simulink model "FuzzyPD_2DOFRobot"  (R2024b)
settings: Solver=FixedStepAuto  StartTime=0.0  StopTime=40.0  FixedStep=0.01  RelTol=1e-3
libraries: neural x58
(part 2 of 2)

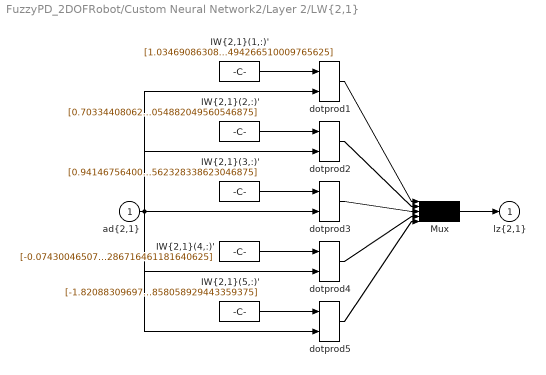
== system FuzzyPD_2DOFRobot/Custom Neural Network2/Layer 2/LW{2,1} ==
  "ad{2,1}" : Inport  PortDimensions=20
      mask Display: e = 0.06;c1 = [120 230 180]/255;c2 = ([120 230 180]+0)/(256+128);c3 = ([120 230 180]+128)/(256+128);patch([0 1 1 0],[0 0 1 1],c1);patch([0 1 1 1-e 1-e 0+e],[0 0 1 1-e 0+e 0+e],c2);patch([0 0 1 1-e 0+e 0+e],[0 1 1 1-e 1-e 0+e],c3);plot([0 1 1 0 0],[0 0 1 1 0]);
  "IW{2,1}(1,:)'" : Constant  Value=[1.034690863083454370752178874681703746318817138671875;0.71478762496765357870032175924279727041721343994140625;-0.9023035135599835054875939022167585790157318115234375;0.433374758147354099957482276295195333659648895263671875;1.2128826774850207659284251349163241684436798095703125;-0.028405390176671818647236023025470785796642303466796875;-0.80937341754777836211331987215089611709117889404296875;-0.545930474311120850217093902756460011005401611328125;0.8748460535361985979108112587709911167621612548828125;0.67782045911715138597486429716809652745723724365234375;-1.0204186771718684045850977781810797750949859619140625;-1.05206299588309892811821555369533598423004150390625;-0.853743879382991455173623762675561010837554931640625;0.860297114781614080669669419876299798488616943359375;1.484280086079977412083508170326240360736846923828125;0.58045414384198534829550908398232422769069671630859375;-0.052367665752894927699845339930107002146542072296142578125;0.2329001374967674120597393994103185832500457763671875;0.772776795739658073358668843866325914859771728515625;-0.58307313814202521573548665401176549494266510009765625]
      mask Display: e = 0.06;c1 = [120 150 230]/255;c2 = ([120 150 230]+0)/383;c3 = ([120 150 230]+128)/383;patch([0 1 1 0],[0 0 1 1],c1);patch([0 1 1 1-e 1-e 0+e],[0 0 1 1-e 0+e 0+e],c2);patch([0 0 1 1-e 0+e 0+e],[0 1 1 1-e 1-e 0+e],c3);plot([0 1 1 0 0],[0 0 1 1 0]);disp('weights');
  "IW{2,1}(2,:)'" : Constant  Value=[0.70334408062744924183817829543841071426868438720703125;-0.53939593820879061514261820775573141872882843017578125;1.137406415460587627563882051617838442325592041015625;-0.4474318401098182906849842765950597822666168212890625;1.6403418277065695551897306359023787081241607666015625;-0.62450917338377631704560144498827867209911346435546875;1.4154537351861751215409412907320074737071990966796875;0.370117096077064722248195494103129021823406219482421875;-1.4599460757945610378527590000885538756847381591796875;1.24160115883402877301477928995154798030853271484375;-0.560063640244826910219444471294991672039031982421875;-0.44157853574027561283088516574935056269168853759765625;0.638904752277584808695110041298903524875640869140625;-0.298521682975893931644151280124788172543048858642578125;1.134156749895475879696959964348934590816497802734375;0.533255671669086606101473080343566834926605224609375;-0.6331474081832733080688058180385269224643707275390625;-1.0542382294758991800875946864834986627101898193359375;-0.43008412156374575818773564606090076267719268798828125;-1.6039047144127873689711805127444677054882049560546875]
      mask Display: e = 0.06;c1 = [120 150 230]/255;c2 = ([120 150 230]+0)/383;c3 = ([120 150 230]+128)/383;patch([0 1 1 0],[0 0 1 1],c1);patch([0 1 1 1-e 1-e 0+e],[0 0 1 1-e 0+e 0+e],c2);patch([0 0 1 1-e 0+e 0+e],[0 1 1 1-e 1-e 0+e],c3);plot([0 1 1 0 0],[0 0 1 1 0]);disp('weights');
  "IW{2,1}(3,:)'" : Constant  Value=[0.94146756400392683783451275303377769887447357177734375;0.4731251034591033022280726072494871914386749267578125;0.352835011006732146565667562754242680966854095458984375;0.83254717249503784604058864715625531971454620361328125;0.3824725814911185128863735371851362287998199462890625;-0.6642082095069279379373483607196249067783355712890625;-0.6011230376676464093321783366263844072818756103515625;0.7943446655054771099457866512238979339599609375;-0.272249257525836119153694880878902040421962738037109375;0.43212706390093968966681359233916737139225006103515625;-0.7383066341177497715619892915128730237483978271484375;-0.366647708417497997235301454566069878637790679931640625;-0.71722827145524148395594465910107828676700592041015625;0.95313490510591158955122637053136713802814483642578125;0.1959390264021163563512573091429658234119415283203125;-0.59216619609386622613556028227321803569793701171875;0.837133704178429471909339554258622229099273681640625;-0.95864630287372076811180932054412551224231719970703125;0.9581049364333307227781233450514264404773712158203125;0.852489248366903762388346876832656562328338623046875]
      mask Display: e = 0.06;c1 = [120 150 230]/255;c2 = ([120 150 230]+0)/383;c3 = ([120 150 230]+128)/383;patch([0 1 1 0],[0 0 1 1],c1);patch([0 1 1 1-e 1-e 0+e],[0 0 1 1-e 0+e 0+e],c2);patch([0 0 1 1-e 0+e 0+e],[0 1 1 1-e 1-e 0+e],c3);plot([0 1 1 0 0],[0 0 1 1 0]);disp('weights');
  "IW{2,1}(4,:)'" : Constant  Value=[-0.07430046507749595019465260747892898507416248321533203125;-0.98614127796260497849090143063222058117389678955078125;0.058465987251093365362208942315191961824893951416015625;0.55693630778370117884179535394650883972644805908203125;0.9257628102854227325479996579815633594989776611328125;-0.72377518289734277256997074800892733037471771240234375;2.023327190999340441379672483890317380428314208984375;-0.330409569161653371427433967255637980997562408447265625;1.2305003744543070443029364469111897051334381103515625;1.409296668044323297408482176251709461212158203125;-0.8464601958773758649812180010485462844371795654296875;-0.15917964775082149575524681495153345167636871337890625;0.022421149902434732437139786043189815245568752288818359375;-1.4635363788993991374098868618602864444255828857421875;0.37541953637812941479978690040297806262969970703125;2.088562987566513928783251685672439634799957275390625;0.47790382938157727199524060779367573559284210205078125;-1.81498933367571613217705817078240215778350830078125;0.337827387873957663000368256689398549497127532958984375;-0.2216054912450064195983401305056759156286716461181640625]
      mask Display: e = 0.06;c1 = [120 150 230]/255;c2 = ([120 150 230]+0)/383;c3 = ([120 150 230]+128)/383;patch([0 1 1 0],[0 0 1 1],c1);patch([0 1 1 1-e 1-e 0+e],[0 0 1 1-e 0+e 0+e],c2);patch([0 0 1 1-e 0+e 0+e],[0 1 1 1-e 1-e 0+e],c3);plot([0 1 1 0 0],[0 0 1 1 0]);disp('weights');
  "IW{2,1}(5,:)'" : Constant  Value=[-1.8208830969722242798525257967412471771240234375;0.69084466334677185894719286807230673730373382568359375;1.122947859773492762514024434494785964488983154296875;-0.317234295989334114107549567052046768367290496826171875;0.62250476604156224080810488885617814958095550537109375;1.6894068695845165795077491566189564764499664306640625;0.288506114882021658107902339907013811171054840087890625;0.58551374156033630935525025051902048289775848388671875;0.6922866926558828293281067089992575347423553466796875;0.6889586364774105131658643585979007184505462646484375;-0.432375825434855531881339629762805998325347900390625;0.097155559921801526446216712429304607212543487548828125;-1.6078115193098370117041895355214364826679229736328125;0.08076992178353738227603031418766477145254611968994140625;0.284325215938594222375712661232682876288890838623046875;2.95425971495564443358716744114644825458526611328125;-1.4133445517274896285897511916118673980236053466796875;-1.9814217989859825852505537113756872713565826416015625;0.98014144968227956411510604084469377994537353515625;-4.094403814209552905367672792635858058929443359375]
      mask Display: e = 0.06;c1 = [120 150 230]/255;c2 = ([120 150 230]+0)/383;c3 = ([120 150 230]+128)/383;patch([0 1 1 0],[0 0 1 1],c1);patch([0 1 1 1-e 1-e 0+e],[0 0 1 1-e 0+e 0+e],c2);patch([0 0 1 1-e 0+e 0+e],[0 1 1 1-e 1-e 0+e],c3);plot([0 1 1 0 0],[0 0 1 1 0]);disp('weights');
  Mux : Mux  Inputs=5
      mask Display: e = 0.06;c1 = [120 150 230]/255;c2 = ([120 150 230]+0)/383;c3 = ([120 150 230]+128)/383;patch([0 1 1 0],[0 0 1 1],c1);patch([0 1 1 1-e 1-e 0+e],[0 0 1 1-e 0+e 0+e],c2);patch([0 0 1 1-e 0+e 0+e],[0 1 1 1-e 1-e 0+e],c3);plot([0 1 1 0 0],[0 0 1 1 0]);disp('Mux');
  dotprod{1..5} (5 alike) : neural/Weight Functions/dotprod
  "lz{2,1}" : Outport
      mask Display: e = 0.06;c1 = [120 230 180]/255;c2 = ([120 230 180]+0)/(256+128);c3 = ([120 230 180]+128)/(256+128);patch([0 1 1 0],[0 0 1 1],c1);patch([0 1 1 1-e 1-e 0+e],[0 0 1 1-e 0+e 0+e],c2);patch([0 0 1 1-e 0+e 0+e],[0 1 1 1-e 1-e 0+e],c3);plot([0 1 1 0 0],[0 0 1 1 0]);
  wires:
  "IW{2,1}(1,:)'"/1 -> dotprod1/1
  "ad{2,1}"/1 -> dotprod1/2, dotprod2/2, dotprod3/2, dotprod4/2, dotprod5/2
  dotprod1/1 -> Mux/1
  "IW{2,1}(2,:)'"/1 -> dotprod2/1
  dotprod2/1 -> Mux/2
  "IW{2,1}(3,:)'"/1 -> dotprod3/1
  dotprod3/1 -> Mux/3
  "IW{2,1}(4,:)'"/1 -> dotprod4/1
  dotprod4/1 -> Mux/4
  "IW{2,1}(5,:)'"/1 -> dotprod5/1
  dotprod5/1 -> Mux/5
  Mux/1 -> "lz{2,1}"/1

== system FuzzyPD_2DOFRobot/Custom Neural Network2/Layer 3/Delays 1 ==
  "p{3}" : Inport  PortDimensions=5
      mask Display: e = 0.06;c1 = [120 230 180]/255;c2 = ([120 230 180]+0)/(256+128);c3 = ([120 230 180]+128)/(256+128);patch([0 1 1 0],[0 0 1 1],c1);patch([0 1 1 1-e 1-e 0+e],[0 0 1 1-e 0+e 0+e],c2);patch([0 0 1 1-e 0+e 0+e],[0 1 1 1-e 1-e 0+e],c3);plot([0 1 1 0 0],[0 0 1 1 0]);
  mux : Mux  Inputs=1
      mask Display: e = 0.06;c1 = [120 150 230]/255;c2 = ([120 150 230]+0)/383;c3 = ([120 150 230]+128)/383;patch([0 1 1 0],[0 0 1 1],c1);patch([0 1 1 1-e 1-e 0+e],[0 0 1 1-e 0+e 0+e],c2);patch([0 0 1 1-e 0+e 0+e],[0 1 1 1-e 1-e 0+e],c3);plot([0 1 1 0 0],[0 0 1 1 0]);disp('Mux')
  "pd{3,2}" : Outport
      mask Display: e = 0.06;c1 = [120 230 180]/255;c2 = ([120 230 180]+0)/(256+128);c3 = ([120 230 180]+128)/(256+128);patch([0 1 1 0],[0 0 1 1],c1);patch([0 1 1 1-e 1-e 0+e],[0 0 1 1-e 0+e 0+e],c2);patch([0 0 1 1-e 0+e 0+e],[0 1 1 1-e 1-e 0+e],c3);plot([0 1 1 0 0],[0 0 1 1 0]);
  wires:
  "p{3}"/1 -> mux/1
  mux/1 -> "pd{3,2}"/1

== system FuzzyPD_2DOFRobot/Custom Neural Network2/Layer 3/LW{3,2} ==
  "ad{3,2}" : Inport  PortDimensions=5
      mask Display: e = 0.06;c1 = [120 230 180]/255;c2 = ([120 230 180]+0)/(256+128);c3 = ([120 230 180]+128)/(256+128);patch([0 1 1 0],[0 0 1 1],c1);patch([0 1 1 1-e 1-e 0+e],[0 0 1 1-e 0+e 0+e],c2);patch([0 0 1 1-e 0+e 0+e],[0 1 1 1-e 1-e 0+e],c3);plot([0 1 1 0 0],[0 0 1 1 0]);
  "IW{3,2}(1,:)'" : Constant  Value=[1.7210370476344756252018441955442540347576141357421875;0.96563713038743392846896540504531003534793853759765625;0.6139936572474160580981106249964796006679534912109375;1.4959984213294006405448044461081735789775848388671875;0.600176864765051387706762398011051118373870849609375]
      mask Display: e = 0.06;c1 = [120 150 230]/255;c2 = ([120 150 230]+0)/383;c3 = ([120 150 230]+128)/383;patch([0 1 1 0],[0 0 1 1],c1);patch([0 1 1 1-e 1-e 0+e],[0 0 1 1-e 0+e 0+e],c2);patch([0 0 1 1-e 0+e 0+e],[0 1 1 1-e 1-e 0+e],c3);plot([0 1 1 0 0],[0 0 1 1 0]);disp('weights');
  Mux : Mux  Inputs=1
      mask Display: e = 0.06;c1 = [120 150 230]/255;c2 = ([120 150 230]+0)/383;c3 = ([120 150 230]+128)/383;patch([0 1 1 0],[0 0 1 1],c1);patch([0 1 1 1-e 1-e 0+e],[0 0 1 1-e 0+e 0+e],c2);patch([0 0 1 1-e 0+e 0+e],[0 1 1 1-e 1-e 0+e],c3);plot([0 1 1 0 0],[0 0 1 1 0]);disp('Mux');
  dotprod1 : neural/Weight Functions/dotprod
  "lz{3,2}" : Outport
      mask Display: e = 0.06;c1 = [120 230 180]/255;c2 = ([120 230 180]+0)/(256+128);c3 = ([120 230 180]+128)/(256+128);patch([0 1 1 0],[0 0 1 1],c1);patch([0 1 1 1-e 1-e 0+e],[0 0 1 1-e 0+e 0+e],c2);patch([0 0 1 1-e 0+e 0+e],[0 1 1 1-e 1-e 0+e],c3);plot([0 1 1 0 0],[0 0 1 1 0]);
  wires:
  "IW{3,2}(1,:)'"/1 -> dotprod1/1
  "ad{3,2}"/1 -> dotprod1/2
  dotprod1/1 -> Mux/1
  Mux/1 -> "lz{3,2}"/1

== system FuzzyPD_2DOFRobot/Custom Neural Network3/Layer 1/Delays 1 ==
  "p{1}" : Inport  PortDimensions=3
      mask Display: e = 0.06;c1 = [120 230 180]/255;c2 = ([120 230 180]+0)/(256+128);c3 = ([120 230 180]+128)/(256+128);patch([0 1 1 0],[0 0 1 1],c1);patch([0 1 1 1-e 1-e 0+e],[0 0 1 1-e 0+e 0+e],c2);patch([0 0 1 1-e 0+e 0+e],[0 1 1 1-e 1-e 0+e],c3);plot([0 1 1 0 0],[0 0 1 1 0]);
  mux : Mux  Inputs=1
      mask Display: e = 0.06;c1 = [120 150 230]/255;c2 = ([120 150 230]+0)/383;c3 = ([120 150 230]+128)/383;patch([0 1 1 0],[0 0 1 1],c1);patch([0 1 1 1-e 1-e 0+e],[0 0 1 1-e 0+e 0+e],c2);patch([0 0 1 1-e 0+e 0+e],[0 1 1 1-e 1-e 0+e],c3);plot([0 1 1 0 0],[0 0 1 1 0]);disp('Mux')
  "pd{1,1}" : Outport
      mask Display: e = 0.06;c1 = [120 230 180]/255;c2 = ([120 230 180]+0)/(256+128);c3 = ([120 230 180]+128)/(256+128);patch([0 1 1 0],[0 0 1 1],c1);patch([0 1 1 1-e 1-e 0+e],[0 0 1 1-e 0+e 0+e],c2);patch([0 0 1 1-e 0+e 0+e],[0 1 1 1-e 1-e 0+e],c3);plot([0 1 1 0 0],[0 0 1 1 0]);
  wires:
  "p{1}"/1 -> mux/1
  mux/1 -> "pd{1,1}"/1

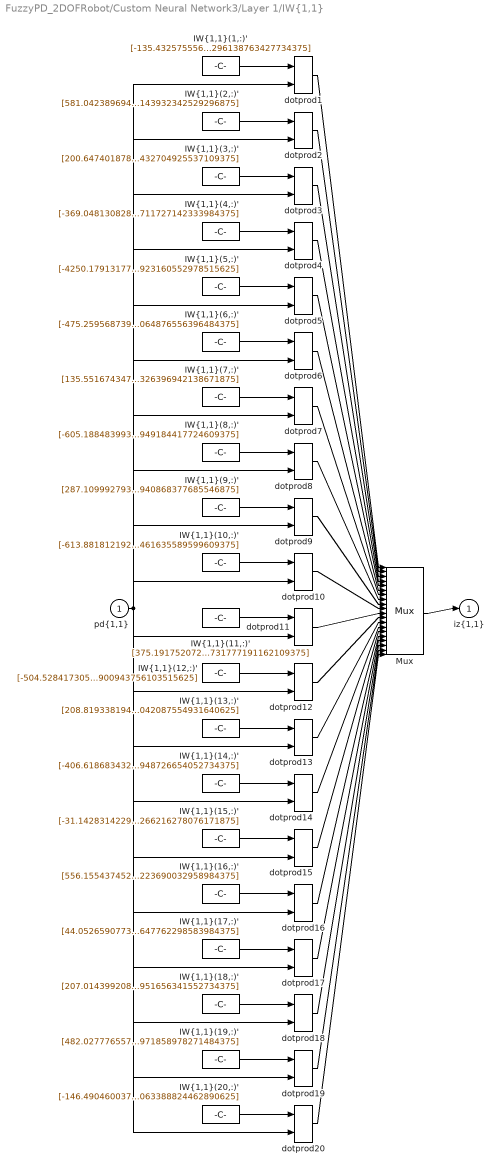
== system FuzzyPD_2DOFRobot/Custom Neural Network3/Layer 1/IW{1,1} ==
  "pd{1,1}" : Inport  PortDimensions=3
      mask Display: e = 0.06;c1 = [120 230 180]/255;c2 = ([120 230 180]+0)/(256+128);c3 = ([120 230 180]+128)/(256+128);patch([0 1 1 0],[0 0 1 1],c1);patch([0 1 1 1-e 1-e 0+e],[0 0 1 1-e 0+e 0+e],c2);patch([0 0 1 1-e 0+e 0+e],[0 1 1 1-e 1-e 0+e],c3);plot([0 1 1 0 0],[0 0 1 1 0]);
  "IW{1,1}(1,:)'" : Constant  Value=[-135.432575556479292799849645234644412994384765625;10.0754622663960358153190099983476102352142333984375;-0.472792983898389473917944769709720276296138763427734375]
      mask Display: e = 0.06;c1 = [120 150 230]/255;c2 = ([120 150 230]+0)/383;c3 = ([120 150 230]+128)/383;patch([0 1 1 0],[0 0 1 1],c1);patch([0 1 1 1-e 1-e 0+e],[0 0 1 1-e 0+e 0+e],c2);patch([0 0 1 1-e 0+e 0+e],[0 1 1 1-e 1-e 0+e],c3);plot([0 1 1 0 0],[0 0 1 1 0]);disp('Weights');
  "IW{1,1}(10,:)'" : Constant  Value=[-613.881812192461666199960745871067047119140625;94.37434568259828893133089877665042877197265625;0.2210466396896054452891888786325580440461635589599609375]
      mask Display: e = 0.06;c1 = [120 150 230]/255;c2 = ([120 150 230]+0)/383;c3 = ([120 150 230]+128)/383;patch([0 1 1 0],[0 0 1 1],c1);patch([0 1 1 1-e 1-e 0+e],[0 0 1 1-e 0+e 0+e],c2);patch([0 0 1 1-e 0+e 0+e],[0 1 1 1-e 1-e 0+e],c3);plot([0 1 1 0 0],[0 0 1 1 0]);disp('Weights');
  "IW{1,1}(11,:)'" : Constant  Value=[375.19175207238521352337556891143321990966796875;-30.256984409509783517933101393282413482666015625;-0.10059679238582529270384924302561557851731777191162109375]
      mask Display: e = 0.06;c1 = [120 150 230]/255;c2 = ([120 150 230]+0)/383;c3 = ([120 150 230]+128)/383;patch([0 1 1 0],[0 0 1 1],c1);patch([0 1 1 1-e 1-e 0+e],[0 0 1 1-e 0+e 0+e],c2);patch([0 0 1 1-e 0+e 0+e],[0 1 1 1-e 1-e 0+e],c3);plot([0 1 1 0 0],[0 0 1 1 0]);disp('Weights');
  "IW{1,1}(12,:)'" : Constant  Value=[-504.52841730549317844634060747921466827392578125;7.89932038819319615186032024212181568145751953125;-0.07291021612746741153987528605284751392900943756103515625]
      mask Display: e = 0.06;c1 = [120 150 230]/255;c2 = ([120 150 230]+0)/383;c3 = ([120 150 230]+128)/383;patch([0 1 1 0],[0 0 1 1],c1);patch([0 1 1 1-e 1-e 0+e],[0 0 1 1-e 0+e 0+e],c2);patch([0 0 1 1-e 0+e 0+e],[0 1 1 1-e 1-e 0+e],c3);plot([0 1 1 0 0],[0 0 1 1 0]);disp('Weights');
  "IW{1,1}(13,:)'" : Constant  Value=[208.819338194989853718652739189565181732177734375;37.72759958928005374900749302469193935394287109375;-0.757522513115136408856642447062768042087554931640625]
      mask Display: e = 0.06;c1 = [120 150 230]/255;c2 = ([120 150 230]+0)/383;c3 = ([120 150 230]+128)/383;patch([0 1 1 0],[0 0 1 1],c1);patch([0 1 1 1-e 1-e 0+e],[0 0 1 1-e 0+e 0+e],c2);patch([0 0 1 1-e 0+e 0+e],[0 1 1 1-e 1-e 0+e],c3);plot([0 1 1 0 0],[0 0 1 1 0]);disp('Weights');
  "IW{1,1}(14,:)'" : Constant  Value=[-406.61868343285050286795012652873992919921875;-24.0765119392089701477743801660835742950439453125;-0.9332100225159842832312051541521213948726654052734375]
      mask Display: e = 0.06;c1 = [120 150 230]/255;c2 = ([120 150 230]+0)/383;c3 = ([120 150 230]+128)/383;patch([0 1 1 0],[0 0 1 1],c1);patch([0 1 1 1-e 1-e 0+e],[0 0 1 1-e 0+e 0+e],c2);patch([0 0 1 1-e 0+e 0+e],[0 1 1 1-e 1-e 0+e],c3);plot([0 1 1 0 0],[0 0 1 1 0]);disp('Weights');
  "IW{1,1}(15,:)'" : Constant  Value=[-31.142831422933721086110381293110549449920654296875;5.93410486604341347316449173376895487308502197265625;0.335283700642425130933332866334239952266216278076171875]
      mask Display: e = 0.06;c1 = [120 150 230]/255;c2 = ([120 150 230]+0)/383;c3 = ([120 150 230]+128)/383;patch([0 1 1 0],[0 0 1 1],c1);patch([0 1 1 1-e 1-e 0+e],[0 0 1 1-e 0+e 0+e],c2);patch([0 0 1 1-e 0+e 0+e],[0 1 1 1-e 1-e 0+e],c3);plot([0 1 1 0 0],[0 0 1 1 0]);disp('Weights');
  "IW{1,1}(16,:)'" : Constant  Value=[556.15543745200511693838052451610565185546875;-62.75604466827012828389342757873237133026123046875;0.98338532426563973753985692383139394223690032958984375]
      mask Display: e = 0.06;c1 = [120 150 230]/255;c2 = ([120 150 230]+0)/383;c3 = ([120 150 230]+128)/383;patch([0 1 1 0],[0 0 1 1],c1);patch([0 1 1 1-e 1-e 0+e],[0 0 1 1-e 0+e 0+e],c2);patch([0 0 1 1-e 0+e 0+e],[0 1 1 1-e 1-e 0+e],c3);plot([0 1 1 0 0],[0 0 1 1 0]);disp('Weights');
  "IW{1,1}(17,:)'" : Constant  Value=[44.05265907730446173218297190032899379730224609375;-23.092237387069513232518147560767829418182373046875;0.94364919863966834068236266830353997647762298583984375]
      mask Display: e = 0.06;c1 = [120 150 230]/255;c2 = ([120 150 230]+0)/383;c3 = ([120 150 230]+128)/383;patch([0 1 1 0],[0 0 1 1],c1);patch([0 1 1 1-e 1-e 0+e],[0 0 1 1-e 0+e 0+e],c2);patch([0 0 1 1-e 0+e 0+e],[0 1 1 1-e 1-e 0+e],c3);plot([0 1 1 0 0],[0 0 1 1 0]);disp('Weights');
  "IW{1,1}(18,:)'" : Constant  Value=[207.014399208383252926068962551653385162353515625;-10.5004037937094931720594104263000190258026123046875;0.049000063312716966856807943031526519916951656341552734375]
      mask Display: e = 0.06;c1 = [120 150 230]/255;c2 = ([120 150 230]+0)/383;c3 = ([120 150 230]+128)/383;patch([0 1 1 0],[0 0 1 1],c1);patch([0 1 1 1-e 1-e 0+e],[0 0 1 1-e 0+e 0+e],c2);patch([0 0 1 1-e 0+e 0+e],[0 1 1 1-e 1-e 0+e],c3);plot([0 1 1 0 0],[0 0 1 1 0]);disp('Weights');
  "IW{1,1}(19,:)'" : Constant  Value=[482.02777655767641817874391563236713409423828125;15.4991899483087092193045464227907359600067138671875;-0.349070997444174524471094400723814032971858978271484375]
      mask Display: e = 0.06;c1 = [120 150 230]/255;c2 = ([120 150 230]+0)/383;c3 = ([120 150 230]+128)/383;patch([0 1 1 0],[0 0 1 1],c1);patch([0 1 1 1-e 1-e 0+e],[0 0 1 1-e 0+e 0+e],c2);patch([0 0 1 1-e 0+e 0+e],[0 1 1 1-e 1-e 0+e],c3);plot([0 1 1 0 0],[0 0 1 1 0]);disp('Weights');
  "IW{1,1}(2,:)'" : Constant  Value=[581.0423896949167783532175235450267791748046875;16.47915141783929726670976378954946994781494140625;0.466023100877216822635062953850138001143932342529296875]
      mask Display: e = 0.06;c1 = [120 150 230]/255;c2 = ([120 150 230]+0)/383;c3 = ([120 150 230]+128)/383;patch([0 1 1 0],[0 0 1 1],c1);patch([0 1 1 1-e 1-e 0+e],[0 0 1 1-e 0+e 0+e],c2);patch([0 0 1 1-e 0+e 0+e],[0 1 1 1-e 1-e 0+e],c3);plot([0 1 1 0 0],[0 0 1 1 0]);disp('Weights');
  "IW{1,1}(20,:)'" : Constant  Value=[-146.490460037200847409621928818523883819580078125;65.6835974049690776155330240726470947265625;0.060311156693250246585424889644855284132063388824462890625]
      mask Display: e = 0.06;c1 = [120 150 230]/255;c2 = ([120 150 230]+0)/383;c3 = ([120 150 230]+128)/383;patch([0 1 1 0],[0 0 1 1],c1);patch([0 1 1 1-e 1-e 0+e],[0 0 1 1-e 0+e 0+e],c2);patch([0 0 1 1-e 0+e 0+e],[0 1 1 1-e 1-e 0+e],c3);plot([0 1 1 0 0],[0 0 1 1 0]);disp('Weights');
  "IW{1,1}(3,:)'" : Constant  Value=[200.647401878155420718030654825270175933837890625;32.5421531128873340321661089546978473663330078125;0.385099895085624088775233531123376451432704925537109375]
      mask Display: e = 0.06;c1 = [120 150 230]/255;c2 = ([120 150 230]+0)/383;c3 = ([120 150 230]+128)/383;patch([0 1 1 0],[0 0 1 1],c1);patch([0 1 1 1-e 1-e 0+e],[0 0 1 1-e 0+e 0+e],c2);patch([0 0 1 1-e 0+e 0+e],[0 1 1 1-e 1-e 0+e],c3);plot([0 1 1 0 0],[0 0 1 1 0]);disp('Weights');
  "IW{1,1}(4,:)'" : Constant  Value=[-369.04813082858544248665566556155681610107421875;2.229120603719899396111259193276055157184600830078125;-0.27087284001736777749869133913307450711727142333984375]
      mask Display: e = 0.06;c1 = [120 150 230]/255;c2 = ([120 150 230]+0)/383;c3 = ([120 150 230]+128)/383;patch([0 1 1 0],[0 0 1 1],c1);patch([0 1 1 1-e 1-e 0+e],[0 0 1 1-e 0+e 0+e],c2);patch([0 0 1 1-e 0+e 0+e],[0 1 1 1-e 1-e 0+e],c3);plot([0 1 1 0 0],[0 0 1 1 0]);disp('Weights');
  "IW{1,1}(5,:)'" : Constant  Value=[-4250.179131777787915780209004878997802734375;21.35109343006629245564909069798886775970458984375;-0.9095295811207879665971631766296923160552978515625]
      mask Display: e = 0.06;c1 = [120 150 230]/255;c2 = ([120 150 230]+0)/383;c3 = ([120 150 230]+128)/383;patch([0 1 1 0],[0 0 1 1],c1);patch([0 1 1 1-e 1-e 0+e],[0 0 1 1-e 0+e 0+e],c2);patch([0 0 1 1-e 0+e 0+e],[0 1 1 1-e 1-e 0+e],c3);plot([0 1 1 0 0],[0 0 1 1 0]);disp('Weights');
  "IW{1,1}(6,:)'" : Constant  Value=[-475.25956873974388372516841627657413482666015625;-38.50212833135109491422554128803312778472900390625;1.2676270783202507885789600550197064876556396484375]
      mask Display: e = 0.06;c1 = [120 150 230]/255;c2 = ([120 150 230]+0)/383;c3 = ([120 150 230]+128)/383;patch([0 1 1 0],[0 0 1 1],c1);patch([0 1 1 1-e 1-e 0+e],[0 0 1 1-e 0+e 0+e],c2);patch([0 0 1 1-e 0+e 0+e],[0 1 1 1-e 1-e 0+e],c3);plot([0 1 1 0 0],[0 0 1 1 0]);disp('Weights');
  "IW{1,1}(7,:)'" : Constant  Value=[135.551674347247882224110071547329425811767578125;-192.756809317032320905127562582492828369140625;0.1987756467040510954813470334556768648326396942138671875]
      mask Display: e = 0.06;c1 = [120 150 230]/255;c2 = ([120 150 230]+0)/383;c3 = ([120 150 230]+128)/383;patch([0 1 1 0],[0 0 1 1],c1);patch([0 1 1 1-e 1-e 0+e],[0 0 1 1-e 0+e 0+e],c2);patch([0 0 1 1-e 0+e 0+e],[0 1 1 1-e 1-e 0+e],c3);plot([0 1 1 0 0],[0 0 1 1 0]);disp('Weights');
  "IW{1,1}(8,:)'" : Constant  Value=[-605.1884839938144295956590212881565093994140625;57.33295746131988579463722999207675457000732421875;-0.161819490490364648049848028676933608949184417724609375]
      mask Display: e = 0.06;c1 = [120 150 230]/255;c2 = ([120 150 230]+0)/383;c3 = ([120 150 230]+128)/383;patch([0 1 1 0],[0 0 1 1],c1);patch([0 1 1 1-e 1-e 0+e],[0 0 1 1-e 0+e 0+e],c2);patch([0 0 1 1-e 0+e 0+e],[0 1 1 1-e 1-e 0+e],c3);plot([0 1 1 0 0],[0 0 1 1 0]);disp('Weights');
  "IW{1,1}(9,:)'" : Constant  Value=[287.1099927932674518160638399422168731689453125;4.393792214334649059992443653754889965057373046875;-0.268791731298118730109081297996453940868377685546875]
      mask Display: e = 0.06;c1 = [120 150 230]/255;c2 = ([120 150 230]+0)/383;c3 = ([120 150 230]+128)/383;patch([0 1 1 0],[0 0 1 1],c1);patch([0 1 1 1-e 1-e 0+e],[0 0 1 1-e 0+e 0+e],c2);patch([0 0 1 1-e 0+e 0+e],[0 1 1 1-e 1-e 0+e],c3);plot([0 1 1 0 0],[0 0 1 1 0]);disp('Weights');
  Mux : Mux  Inputs=20
      mask Display: e = 0.06;c1 = [120 150 230]/255;c2 = ([120 150 230]+0)/383;c3 = ([120 150 230]+128)/383;patch([0 1 1 0],[0 0 1 1],c1);patch([0 1 1 1-e 1-e 0+e],[0 0 1 1-e 0+e 0+e],c2);patch([0 0 1 1-e 0+e 0+e],[0 1 1 1-e 1-e 0+e],c3);plot([0 1 1 0 0],[0 0 1 1 0]);disp('Mux');
  dotprod{1..20} (20 alike) : neural/Weight Functions/dotprod
  "iz{1,1}" : Outport
      mask Display: e = 0.06;c1 = [120 230 180]/255;c2 = ([120 230 180]+0)/(256+128);c3 = ([120 230 180]+128)/(256+128);patch([0 1 1 0],[0 0 1 1],c1);patch([0 1 1 1-e 1-e 0+e],[0 0 1 1-e 0+e 0+e],c2);patch([0 0 1 1-e 0+e 0+e],[0 1 1 1-e 1-e 0+e],c3);plot([0 1 1 0 0],[0 0 1 1 0]);
  wires:
  "IW{1,1}(1,:)'"/1 -> dotprod1/1
  "pd{1,1}"/1 -> dotprod1/2, dotprod2/2, dotprod3/2, dotprod4/2, dotprod5/2, dotprod6/2, dotprod7/2, dotprod8/2, dotprod9/2, dotprod10/2, dotprod11/2, dotprod12/2, dotprod13/2, dotprod14/2, dotprod15/2, dotprod16/2, dotprod17/2, dotprod18/2, dotprod19/2, dotprod20/2
  dotprod1/1 -> Mux/1
  "IW{1,1}(2,:)'"/1 -> dotprod2/1
  dotprod2/1 -> Mux/2
  "IW{1,1}(3,:)'"/1 -> dotprod3/1
  dotprod3/1 -> Mux/3
  "IW{1,1}(4,:)'"/1 -> dotprod4/1
  dotprod4/1 -> Mux/4
  "IW{1,1}(5,:)'"/1 -> dotprod5/1
  dotprod5/1 -> Mux/5
  "IW{1,1}(6,:)'"/1 -> dotprod6/1
  dotprod6/1 -> Mux/6
  "IW{1,1}(7,:)'"/1 -> dotprod7/1
  dotprod7/1 -> Mux/7
  "IW{1,1}(8,:)'"/1 -> dotprod8/1
  dotprod8/1 -> Mux/8
  "IW{1,1}(9,:)'"/1 -> dotprod9/1
  dotprod9/1 -> Mux/9
  "IW{1,1}(10,:)'"/1 -> dotprod10/1
  dotprod10/1 -> Mux/10
  "IW{1,1}(11,:)'"/1 -> dotprod11/1
  dotprod11/1 -> Mux/11
  "IW{1,1}(12,:)'"/1 -> dotprod12/1
  dotprod12/1 -> Mux/12
  "IW{1,1}(13,:)'"/1 -> dotprod13/1
  dotprod13/1 -> Mux/13
  "IW{1,1}(14,:)'"/1 -> dotprod14/1
  dotprod14/1 -> Mux/14
  "IW{1,1}(15,:)'"/1 -> dotprod15/1
  dotprod15/1 -> Mux/15
  "IW{1,1}(16,:)'"/1 -> dotprod16/1
  dotprod16/1 -> Mux/16
  "IW{1,1}(17,:)'"/1 -> dotprod17/1
  dotprod17/1 -> Mux/17
  "IW{1,1}(18,:)'"/1 -> dotprod18/1
  dotprod18/1 -> Mux/18
  "IW{1,1}(19,:)'"/1 -> dotprod19/1
  dotprod19/1 -> Mux/19
  "IW{1,1}(20,:)'"/1 -> dotprod20/1
  dotprod20/1 -> Mux/20
  Mux/1 -> "iz{1,1}"/1

== system FuzzyPD_2DOFRobot/Custom Neural Network3/Layer 2/Delays 1 ==
  "p{2}" : Inport  PortDimensions=20
      mask Display: e = 0.06;c1 = [120 230 180]/255;c2 = ([120 230 180]+0)/(256+128);c3 = ([120 230 180]+128)/(256+128);patch([0 1 1 0],[0 0 1 1],c1);patch([0 1 1 1-e 1-e 0+e],[0 0 1 1-e 0+e 0+e],c2);patch([0 0 1 1-e 0+e 0+e],[0 1 1 1-e 1-e 0+e],c3);plot([0 1 1 0 0],[0 0 1 1 0]);
  mux : Mux  Inputs=1
      mask Display: e = 0.06;c1 = [120 150 230]/255;c2 = ([120 150 230]+0)/383;c3 = ([120 150 230]+128)/383;patch([0 1 1 0],[0 0 1 1],c1);patch([0 1 1 1-e 1-e 0+e],[0 0 1 1-e 0+e 0+e],c2);patch([0 0 1 1-e 0+e 0+e],[0 1 1 1-e 1-e 0+e],c3);plot([0 1 1 0 0],[0 0 1 1 0]);disp('Mux')
  "pd{2,1}" : Outport
      mask Display: e = 0.06;c1 = [120 230 180]/255;c2 = ([120 230 180]+0)/(256+128);c3 = ([120 230 180]+128)/(256+128);patch([0 1 1 0],[0 0 1 1],c1);patch([0 1 1 1-e 1-e 0+e],[0 0 1 1-e 0+e 0+e],c2);patch([0 0 1 1-e 0+e 0+e],[0 1 1 1-e 1-e 0+e],c3);plot([0 1 1 0 0],[0 0 1 1 0]);
  wires:
  "p{2}"/1 -> mux/1
  mux/1 -> "pd{2,1}"/1

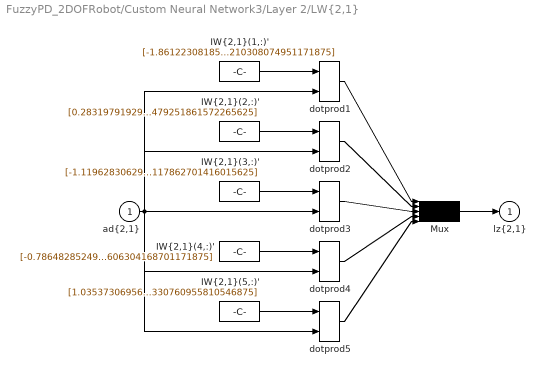
== system FuzzyPD_2DOFRobot/Custom Neural Network3/Layer 2/LW{2,1} ==
  "ad{2,1}" : Inport  PortDimensions=20
      mask Display: e = 0.06;c1 = [120 230 180]/255;c2 = ([120 230 180]+0)/(256+128);c3 = ([120 230 180]+128)/(256+128);patch([0 1 1 0],[0 0 1 1],c1);patch([0 1 1 1-e 1-e 0+e],[0 0 1 1-e 0+e 0+e],c2);patch([0 0 1 1-e 0+e 0+e],[0 1 1 1-e 1-e 0+e],c3);plot([0 1 1 0 0],[0 0 1 1 0]);
  "IW{2,1}(1,:)'" : Constant  Value=[-1.8612230818564337031517652576440013945102691650390625;-1.071564998167807925000261093373410403728485107421875;-3.23871240049929287607710648444481194019317626953125;-1.6828789835814330633212421162170358002185821533203125;2.6751370085307062396395849646069109439849853515625;0.556260594094869720294127546367235481739044189453125;0.25208317227902654611426669362117536365985870361328125;0.07264863219442900532651918865667539648711681365966796875;6.4659008917615761191655110451392829418182373046875;-0.406095293463918205478790923734777607023715972900390625;-1.22624806521601659170528364484198391437530517578125;1.39698201299491842064526281319558620452880859375;-0.81000316067316668888764752409770153462886810302734375;3.788956823273356366854613952455110847949981689453125;-1.2830479721001337711783207851112820208072662353515625;2.508688006071150056186525034718215465545654296875;-3.257453779755907330439868019311688840389251708984375;0.44446320017796636658857778456876985728740692138671875;-6.52708449968819603981273758108727633953094482421875;1.09821961659860534155086497776210308074951171875]
      mask Display: e = 0.06;c1 = [120 150 230]/255;c2 = ([120 150 230]+0)/383;c3 = ([120 150 230]+128)/383;patch([0 1 1 0],[0 0 1 1],c1);patch([0 1 1 1-e 1-e 0+e],[0 0 1 1-e 0+e 0+e],c2);patch([0 0 1 1-e 0+e 0+e],[0 1 1 1-e 1-e 0+e],c3);plot([0 1 1 0 0],[0 0 1 1 0]);disp('weights');
  "IW{2,1}(2,:)'" : Constant  Value=[0.28319791929440130129336239406256936490535736083984375;-0.54250982965030658533578389324247837066650390625;-3.126259997898063858201567200012505054473876953125;1.26338281147565378859098927932791411876678466796875;0.45086880669833195867113317945040762424468994140625;-1.2801619837682902680597862854483537375926971435546875;-0.478054406947438781383397099489229731261730194091796875;1.3260739172309292666085411838139407336711883544921875;-8.6646189148814425351474710623733699321746826171875;-0.46726354027927907708317434298805892467498779296875;-1.0161450348850549207924132133484818041324615478515625;-1.3140327429924634206059863572590984404087066650390625;-1.5160928295874638305207326993695460259914398193359375;1.874957650721968516194237963645718991756439208984375;-0.73377471724072440562025576582527719438076019287109375;0.138128365176629352983894705175771377980709075927734375;-1.714395084681551661986986800911836326122283935546875;-0.8874257838450929636309183479170314967632293701171875;-2.002363192255565582655663092737086117267608642578125;-1.509434193550879488299187869415618479251861572265625]
      mask Display: e = 0.06;c1 = [120 150 230]/255;c2 = ([120 150 230]+0)/383;c3 = ([120 150 230]+128)/383;patch([0 1 1 0],[0 0 1 1],c1);patch([0 1 1 1-e 1-e 0+e],[0 0 1 1-e 0+e 0+e],c2);patch([0 0 1 1-e 0+e 0+e],[0 1 1 1-e 1-e 0+e],c3);plot([0 1 1 0 0],[0 0 1 1 0]);disp('weights');
  "IW{2,1}(3,:)'" : Constant  Value=[-1.1196283062952681053303649605368264019489288330078125;2.879738270594077942376998180407099425792694091796875;0.1405512492790717271606837357467156834900379180908203125;-0.987438767336694223075710397097282111644744873046875;0.66943456196333561702971337581402622163295745849609375;0.44317065063744809361168108807760290801525115966796875;0.7693690148018388352824104003957472741603851318359375;-0.240872143271876837378187019567121751606464385986328125;0.212958332877191180987352936426759697496891021728515625;0.3067548871261325249548690408119000494480133056640625;0.88040201213680535641259439216810278594493865966796875;0.562644161332072290093719857395626604557037353515625;-1.084563267733756664057409579982049763202667236328125;0.37957535576649714670338653377257287502288818359375;0.044349003777790392544222441983947646804153919219970703125;0.0262761870024459907868585872847688733600080013275146484375;-0.388668181877419749437052587381913326680660247802734375;-1.380387200777627665360114406212233006954193115234375;0.12919389093648570021599653045996092259883880615234375;5.38096448750756994883204242796637117862701416015625]
      mask Display: e = 0.06;c1 = [120 150 230]/255;c2 = ([120 150 230]+0)/383;c3 = ([120 150 230]+128)/383;patch([0 1 1 0],[0 0 1 1],c1);patch([0 1 1 1-e 1-e 0+e],[0 0 1 1-e 0+e 0+e],c2);patch([0 0 1 1-e 0+e 0+e],[0 1 1 1-e 1-e 0+e],c3);plot([0 1 1 0 0],[0 0 1 1 0]);disp('weights');
  "IW{2,1}(4,:)'" : Constant  Value=[-0.78648285249726057610786256191204302012920379638671875;-1.9714725331353177839588397546322084963321685791015625;-0.09075520380047559509950616529749822802841663360595703125;-1.1227593442808856405434880798566155135631561279296875;-2.82112594910226821554033449501730501651763916015625;0.76872070689084692762804706944734789431095123291015625;0.69398273938297727614354926117812283337116241455078125;1.755413184869441867164141513057984411716461181640625;5.09412128049174572907986657810397446155548095703125;-1.7064902953390423956392396576120518147945404052734375;2.0219614873711737601524873753078281879425048828125;-1.1511360158621288807268001619377173483371734619140625;0.8982685532896945712622027713223360478878021240234375;-1.6322420219143822794904963302542455494403839111328125;0.64102724757909468333849645205191336572170257568359375;1.040596986943088442245652913697995245456695556640625;0.464893266486310630103417906866525299847126007080078125;-0.1474689639994558321145490253911702893674373626708984375;2.017670497708806909287204689462669193744659423828125;-0.1000985734520889181009550839007715694606304168701171875]
      mask Display: e = 0.06;c1 = [120 150 230]/255;c2 = ([120 150 230]+0)/383;c3 = ([120 150 230]+128)/383;patch([0 1 1 0],[0 0 1 1],c1);patch([0 1 1 1-e 1-e 0+e],[0 0 1 1-e 0+e 0+e],c2);patch([0 0 1 1-e 0+e 0+e],[0 1 1 1-e 1-e 0+e],c3);plot([0 1 1 0 0],[0 0 1 1 0]);disp('weights');
  "IW{2,1}(5,:)'" : Constant  Value=[1.035373069568306103604982126853428781032562255859375;1.046618128101016065301109847496263682842254638671875;-0.316915385107774116857370927391457371413707733154296875;2.504064611485200320117883165949024260044097900390625;-1.1147430392958435074746148529811762273311614990234375;0.90660327991771882949478822411037981510162353515625;1.513934544792630010334733015042729675769805908203125;-1.6807830070619711460011558301630429923534393310546875;2.536628645430968997942500209319405257701873779296875;-0.56775998776683878066506849791039712727069854736328125;1.3403330777112139049478400920634157955646514892578125;-3.11147636937384053368305103504098951816558837890625;-1.3754153770593677830191836619633249938488006591796875;-1.6175075972446271155291697141365148127079010009765625;2.33429463679302617862276747473515570163726806640625;3.670223097440406423430658833240158855915069580078125;-0.52797349334209953131136217052699066698551177978515625;1.2137995413191602356306475485325790941715240478515625;1.2802832963744312788634260869002901017665863037109375;-1.5615939650356362999872317232075147330760955810546875]
      mask Display: e = 0.06;c1 = [120 150 230]/255;c2 = ([120 150 230]+0)/383;c3 = ([120 150 230]+128)/383;patch([0 1 1 0],[0 0 1 1],c1);patch([0 1 1 1-e 1-e 0+e],[0 0 1 1-e 0+e 0+e],c2);patch([0 0 1 1-e 0+e 0+e],[0 1 1 1-e 1-e 0+e],c3);plot([0 1 1 0 0],[0 0 1 1 0]);disp('weights');
  Mux : Mux  Inputs=5
      mask Display: e = 0.06;c1 = [120 150 230]/255;c2 = ([120 150 230]+0)/383;c3 = ([120 150 230]+128)/383;patch([0 1 1 0],[0 0 1 1],c1);patch([0 1 1 1-e 1-e 0+e],[0 0 1 1-e 0+e 0+e],c2);patch([0 0 1 1-e 0+e 0+e],[0 1 1 1-e 1-e 0+e],c3);plot([0 1 1 0 0],[0 0 1 1 0]);disp('Mux');
  dotprod{1..5} (5 alike) : neural/Weight Functions/dotprod
  "lz{2,1}" : Outport
      mask Display: e = 0.06;c1 = [120 230 180]/255;c2 = ([120 230 180]+0)/(256+128);c3 = ([120 230 180]+128)/(256+128);patch([0 1 1 0],[0 0 1 1],c1);patch([0 1 1 1-e 1-e 0+e],[0 0 1 1-e 0+e 0+e],c2);patch([0 0 1 1-e 0+e 0+e],[0 1 1 1-e 1-e 0+e],c3);plot([0 1 1 0 0],[0 0 1 1 0]);
  wires:
  "IW{2,1}(1,:)'"/1 -> dotprod1/1
  "ad{2,1}"/1 -> dotprod1/2, dotprod2/2, dotprod3/2, dotprod4/2, dotprod5/2
  dotprod1/1 -> Mux/1
  "IW{2,1}(2,:)'"/1 -> dotprod2/1
  dotprod2/1 -> Mux/2
  "IW{2,1}(3,:)'"/1 -> dotprod3/1
  dotprod3/1 -> Mux/3
  "IW{2,1}(4,:)'"/1 -> dotprod4/1
  dotprod4/1 -> Mux/4
  "IW{2,1}(5,:)'"/1 -> dotprod5/1
  dotprod5/1 -> Mux/5
  Mux/1 -> "lz{2,1}"/1

== system FuzzyPD_2DOFRobot/Custom Neural Network3/Layer 3/Delays 1 ==
  "p{3}" : Inport  PortDimensions=5
      mask Display: e = 0.06;c1 = [120 230 180]/255;c2 = ([120 230 180]+0)/(256+128);c3 = ([120 230 180]+128)/(256+128);patch([0 1 1 0],[0 0 1 1],c1);patch([0 1 1 1-e 1-e 0+e],[0 0 1 1-e 0+e 0+e],c2);patch([0 0 1 1-e 0+e 0+e],[0 1 1 1-e 1-e 0+e],c3);plot([0 1 1 0 0],[0 0 1 1 0]);
  mux : Mux  Inputs=1
      mask Display: e = 0.06;c1 = [120 150 230]/255;c2 = ([120 150 230]+0)/383;c3 = ([120 150 230]+128)/383;patch([0 1 1 0],[0 0 1 1],c1);patch([0 1 1 1-e 1-e 0+e],[0 0 1 1-e 0+e 0+e],c2);patch([0 0 1 1-e 0+e 0+e],[0 1 1 1-e 1-e 0+e],c3);plot([0 1 1 0 0],[0 0 1 1 0]);disp('Mux')
  "pd{3,2}" : Outport
      mask Display: e = 0.06;c1 = [120 230 180]/255;c2 = ([120 230 180]+0)/(256+128);c3 = ([120 230 180]+128)/(256+128);patch([0 1 1 0],[0 0 1 1],c1);patch([0 1 1 1-e 1-e 0+e],[0 0 1 1-e 0+e 0+e],c2);patch([0 0 1 1-e 0+e 0+e],[0 1 1 1-e 1-e 0+e],c3);plot([0 1 1 0 0],[0 0 1 1 0]);
  wires:
  "p{3}"/1 -> mux/1
  mux/1 -> "pd{3,2}"/1

== system FuzzyPD_2DOFRobot/Custom Neural Network3/Layer 3/LW{3,2} ==
  "ad{3,2}" : Inport  PortDimensions=5
      mask Display: e = 0.06;c1 = [120 230 180]/255;c2 = ([120 230 180]+0)/(256+128);c3 = ([120 230 180]+128)/(256+128);patch([0 1 1 0],[0 0 1 1],c1);patch([0 1 1 1-e 1-e 0+e],[0 0 1 1-e 0+e 0+e],c2);patch([0 0 1 1-e 0+e 0+e],[0 1 1 1-e 1-e 0+e],c3);plot([0 1 1 0 0],[0 0 1 1 0]);
  "IW{3,2}(1,:)'" : Constant  Value=[-4.97297437042459389289206228568218648433685302734375;-0.495560990512270593821853026383905671536922454833984375;7.42637078650991799833036566269584000110626220703125;2.90542624297832130508822956471703946590423583984375;3.2302881377498646742196797276847064495086669921875]
      mask Display: e = 0.06;c1 = [120 150 230]/255;c2 = ([120 150 230]+0)/383;c3 = ([120 150 230]+128)/383;patch([0 1 1 0],[0 0 1 1],c1);patch([0 1 1 1-e 1-e 0+e],[0 0 1 1-e 0+e 0+e],c2);patch([0 0 1 1-e 0+e 0+e],[0 1 1 1-e 1-e 0+e],c3);plot([0 1 1 0 0],[0 0 1 1 0]);disp('weights');
  Mux : Mux  Inputs=1
      mask Display: e = 0.06;c1 = [120 150 230]/255;c2 = ([120 150 230]+0)/383;c3 = ([120 150 230]+128)/383;patch([0 1 1 0],[0 0 1 1],c1);patch([0 1 1 1-e 1-e 0+e],[0 0 1 1-e 0+e 0+e],c2);patch([0 0 1 1-e 0+e 0+e],[0 1 1 1-e 1-e 0+e],c3);plot([0 1 1 0 0],[0 0 1 1 0]);disp('Mux');
  dotprod1 : neural/Weight Functions/dotprod
  "lz{3,2}" : Outport
      mask Display: e = 0.06;c1 = [120 230 180]/255;c2 = ([120 230 180]+0)/(256+128);c3 = ([120 230 180]+128)/(256+128);patch([0 1 1 0],[0 0 1 1],c1);patch([0 1 1 1-e 1-e 0+e],[0 0 1 1-e 0+e 0+e],c2);patch([0 0 1 1-e 0+e 0+e],[0 1 1 1-e 1-e 0+e],c3);plot([0 1 1 0 0],[0 0 1 1 0]);
  wires:
  "IW{3,2}(1,:)'"/1 -> dotprod1/1
  "ad{3,2}"/1 -> dotprod1/2
  dotprod1/1 -> Mux/1
  Mux/1 -> "lz{3,2}"/1

== matlab function FuzzyPD_2DOFRobot/Subsystem1/ROBOT_Arm2DOF ==
  data: tor1 input; the1_dd output; tor2 input; the1 input; the2 input; the1_d input; the2_d input; the2_dd output
function [the1_dd, the2_dd] = fcn(tor1, tor2, the1, the2, the1_d, the2_d)
%#codegen
% Modèle dynamique du bras robotique 2-DoF
% Entrées: torques (Nm), positions (rad), vitesses (rad/s)
% Sorties: accélérations (rad/s²)

% --- Paramètres physiques ---
J1 = 0.05;      % Moment d'inertie joint 1 [kg·m²]
J2 = 0.05;      % Moment d'inertie joint 2 [kg·m²]
m1 = 1.0;       % Masse lien 1 [kg]
m2 = 1.0;       % Masse lien 2 [kg]
l1 = 1.0;       % Longueur lien 1 [m]
l2 = 1.0;       % Longueur lien 2 [m]
lc1 = 0.4;      % Distance CG lien 1 [m]
lc2 = 0.4;      % Distance CG lien 2 [m]
g = 9.81;       % Gravité [m/s²]

% --- Calculs intermédiaires ---
c2 = cos(the2);   % cos(theta2)
s2 = sin(the2);   % sin(theta2)
c12 = cos(the1 + the2);  % cos(theta1 + theta2)

% --- Matrice d'inertie M(theta) ---
% Élément M11
M11 = J1 + J2 + m1*lc1^2 + m2*(l1^2 + lc2^2 + 2*l1*lc2*c2);

% Élément M12 = M21
M12 = J2 + m2*(lc2^2 + l1*lc2*c2);

% Élément M22
M22 = J2 + m2*lc2^2;

% Construction de la matrice M
M = [M11, M12;
     M12, M22];  % Car M21 = M12 (matrice symétrique)

% --- Matrice de Coriolis/Centrifuge C(theta, theta_dot) ---
% Terme -m2*l1*lc2*s2
h = -m2*l1*lc2*s2;

% Construction de la matrice C
% Note: C est une matrice 2x2 selon la formule du manuel
C = [h*the2_d,     h*(the1_d + the2_d);
     -h*the1_d,    0];

% --- Vecteur de gravité G(theta) ---
G1 = (m1 + m2)*g*lc1*cos(the1) + m2*g*lc2*c12;
G2 = m2*g*lc2*c12;

G = [G1; G2];

% --- Vecteur d'état (vitesses) ---
theta_dot = [the1_d; the2_d];

% --- Calcul de l'accélération ---
% Équation: M * theta_ddot = tau - C * theta_dot - G
% Donc: theta_ddot = inv(M) * (tau - C*theta_dot - G)

tau = [tor1; tor2];  % Vecteur de couples

% Calcul du terme droit de l'équation
right_side = tau - C*theta_dot - G;

% Résolution pour theta_ddot (accélérations)
% Utilisation de l'opérateur backslash (plus stable que inv(M))
theta_ddot = M \ right_side;

% --- Extraction des sorties ---
the1_dd = theta_ddot(1);
the2_dd = theta_ddot(2);

end
